simulink model "Launch_controlV1_a"  (R2015a)
settings: Solver=ode3  StartTime=0.0  StopTime=inf  FixedStep=0.001  RelTol=1e-3
undefined symbols (not defined in the file or in its folder): DiscIntNeverNeededParam, Ts
libraries: simulink x3
settings Model: CovModelRefEnable=off  Creator=Sven-VDR  LastModifiedBy=Sven-VDR
settings DataIOCC: SaveFormat=Dataset
settings HardwareCC: ProdBitPerPointer=64  ProdLargestAtomicFloat=Float  ProdIntDivRoundTo=Zero  ProdEndianess=LittleEndian  ProdHWDeviceType=Specified
settings GRTTargetCC: GeneratePreprocessorConditionals=Use local settings

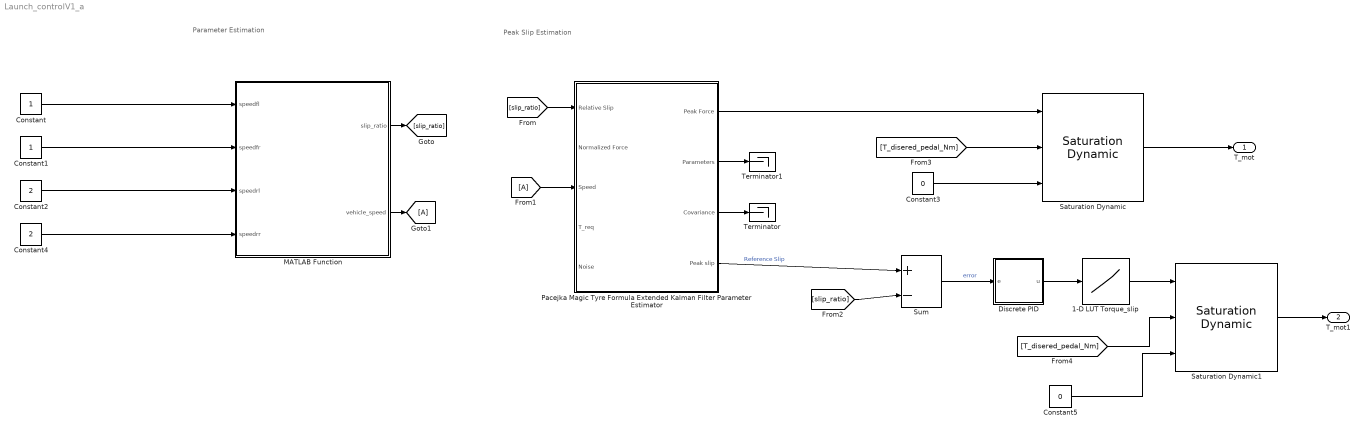
== system Launch_controlV1_a ==
  note: Peak Slip Estimation
  note: Parameter Estimation
  1-D LUT Torque_slip : Lookup_n-D  NumberOfTableDimensions=1  BreakpointsForDimension1=[-5:5]  Table=tanh([-5:5])  InternalRulePriority=Speed  RndMeth=Simplest  InputSameDT=on
  Constant : Constant
  Constant1 : Constant
  Constant2 : Constant  Value=2
  Constant3 : Constant  Value=0
  Constant4 : Constant  Value=2
  Constant5 : Constant  Value=0
  Discrete PID : Subsystem
  MATLAB Function : MATLAB Function  TreatAsAtomicUnit=on
      settings: PermitHierarchicalResolution=ParametersOnly
  Pacejka Magic Tyre Formula Extended Kalman Filter Parameter Estimator : Subsystem
  Saturation Dynamic : simulink/Discontinuities/Saturation Dynamic  OutMin=[]  OutMax=[]  OutDataTypeStr=Inherit: Same as second input  OutDataType=fixdt(1, 16)  OutScaling=2^-10  DoSatur=off
  Saturation Dynamic1 : simulink/Discontinuities/Saturation Dynamic  OutMin=[]  OutMax=[]  OutDataTypeStr=Inherit: Same as second input  OutDataType=fixdt(1, 16)  OutScaling=2^-10  DoSatur=off
  Sum : Sum  Inputs=+|-
  Terminator : Terminator
  Terminator1 : Terminator
  T_mot : Outport
  T_mot1 : Outport  Port=2
  wires:
  Constant2/1 -> MATLAB Function/3(speedrl)
  Constant/1 -> MATLAB Function/1(speedfl)
  Constant4/1 -> MATLAB Function/4(speedrr)
  Constant1/1 -> MATLAB Function/2(speedfr)
  MATLAB Function/1(slip_ratio) -> [slip_ratio]
  MATLAB Function/2(vehicle_speed) -> [A]
  [slip_ratio] -> Pacejka Magic Tyre Formula Extended Kalman Filter Parameter Estimator/1(Relative Slip)
  [A] -> Pacejka Magic Tyre Formula Extended Kalman Filter Parameter Estimator/3(Speed)
  Pacejka Magic Tyre Formula Extended Kalman Filter Parameter Estimator/4(Peak slip) -> Sum/1  "Reference Slip"
  Pacejka Magic Tyre Formula Extended Kalman Filter Parameter Estimator/3(Covariance) -> Terminator/1
  Pacejka Magic Tyre Formula Extended Kalman Filter Parameter Estimator/2(Parameters) -> Terminator1/1
  Sum/1 -> Discrete PID/1("e ")  "error"
  [slip_ratio] -> Sum/2
  Constant3/1 -> Saturation Dynamic/3
  Pacejka Magic Tyre Formula Extended Kalman Filter Parameter Estimator/1(Peak Force) -> Saturation Dynamic/1
  [T_disered_pedal_Nm] -> Saturation Dynamic/2
  Saturation Dynamic/1 -> T_mot/1
  Discrete PID/1(u) -> 1-D LUT Torque_slip/1
  1-D LUT Torque_slip/1 -> Saturation Dynamic1/1
  [T_disered_pedal_Nm] -> Saturation Dynamic1/2
  Constant5/1 -> Saturation Dynamic1/3
  Saturation Dynamic1/1 -> T_mot1/1

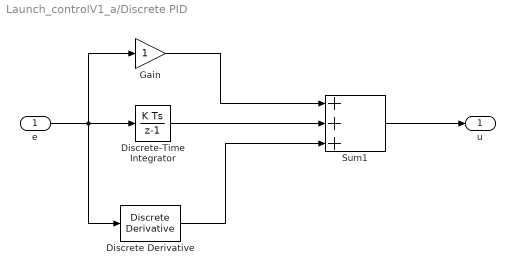
== system Launch_controlV1_a/Discrete PID ==
  "e " : Inport
  Discrete Derivative : simulink/Discrete/Discrete Derivative  gainval=1.0  ICPrevScaledInput=0.0  InputProcessing=Inherited  OutMin=[]  OutMax=[]  OutDataType=fixdt(1, 16)  OutScaling=2^-10  DoSatur=off
  Discrete-Time Integrator : DiscreteIntegrator  InitialConditionSetting=State (most efficient)  ICPrevOutput=DiscIntNeverNeededParam  ICPrevScaledInput=DiscIntNeverNeededParam
  Gain : Gain
  Sum1 : Sum  Inputs=+|+|+
  u : Outport
  wires:
  "e "/1 -> Discrete Derivative/1, Discrete-Time Integrator/1, Gain/1
  Sum1/1 -> u/1
  Discrete-Time Integrator/1 -> Sum1/2
  Gain/1 -> Sum1/1
  Discrete Derivative/1 -> Sum1/3

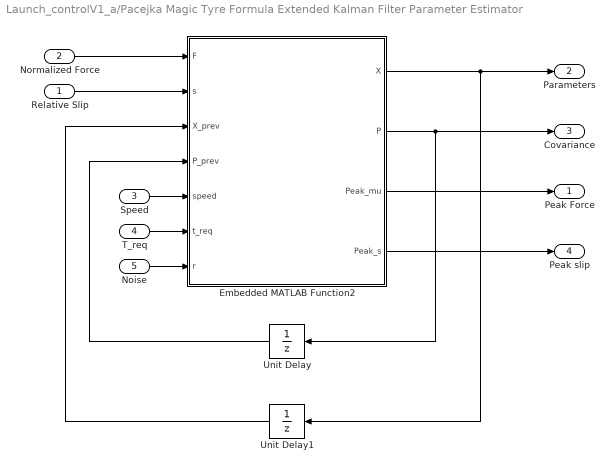
== system Launch_controlV1_a/Pacejka Magic Tyre Formula Extended Kalman Filter Parameter Estimator ==
  Relative Slip : Inport
  Normalized Force : Inport  Port=2
  Speed : Inport  Port=3
  T_req : Inport  Port=4
  Noise : Inport  Port=5
  Embedded MATLAB Function2 : MATLAB Function  TreatAsAtomicUnit=on
      settings: PermitHierarchicalResolution=ParametersOnly
  Unit Delay : UnitDelay  InitialCondition=[1 0 0 0 0; 0 3 0 0 0; 0 0 3 0 0; 0 0 0 0.5 0; 0 0 0 0 5]  SampleTime=Ts
  Unit Delay1 : UnitDelay  InitialCondition=[15;2;2;0.9;0]  SampleTime=Ts
  Peak Force : Outport
  Parameters : Outport  Port=2
  Covariance : Outport  Port=3
  Peak slip : Outport  Port=4
  wires:
  Embedded MATLAB Function2/2(P) -> Covariance/1, Unit Delay/1
  Unit Delay/1 -> Embedded MATLAB Function2/4(P_prev)
  Embedded MATLAB Function2/1(X) -> Parameters/1, Unit Delay1/1
  Unit Delay1/1 -> Embedded MATLAB Function2/3(X_prev)
  Normalized Force/1 -> Embedded MATLAB Function2/1(F)
  Relative Slip/1 -> Embedded MATLAB Function2/2(s)
  Embedded MATLAB Function2/3(Peak_mu) -> Peak Force/1
  Speed/1 -> Embedded MATLAB Function2/5(speed)
  T_req/1 -> Embedded MATLAB Function2/6(t_req)
  Noise/1 -> Embedded MATLAB Function2/7(r)
  Embedded MATLAB Function2/4(Peak_s) -> Peak slip/1

== matlab function Launch_controlV1_a/MATLAB Function ==
  data: speedfl input; slip_ratio output; speedfr input; speedrl input; speedrr input; vehicle_speed output
function [slip_ratio, vehicle_speed]=Launch_slip_calc(speedfl,speedfr,speedrl,speedrr)
%Calculates the wheel slip ratio
rwheel=0.254; %m

Rotspeed_front=(speedfl+speedfr)/2;
Rotspeed_rear = max(speedrl,speedrr);

vehicle_speed=Rotspeed_front*rwheel;

slip_ratio=(1-vehicle_speed/(rwheel*Rotspeed_rear));

if slip_ratio<0
    slip_ratio=0;
end

end

== matlab function Launch_controlV1_a/Pacejka Magic Tyre Formula Extended Kalman Filter Parameter Estimator/Embedded MATLAB Function2 ==
  data: F input; s input; X_prev input; X output; P_prev input; P output; Peak_mu output; speed input; t_req input; r input; Peak_s output
function [X,P,Peak_mu,Peak_s]= Magic_Formula(F,s,X_prev,P_prev,speed,t_req,r)
    
% Initialization

X = X_prev;
P = P_prev;

% Kalman Filter Algorithm (Pacejka Magic Formula)
% State X consists of B, C, D, E, Sv, Sh (in this order)

B = X(1,1);
C = X(2,1);
D = X(3,1);
E = X(4,1);
Sh = X(5,1);

% Noise
%r = [0.01 0; 0 0.1];

if (s >= 0.02 && s <= 0.10 && F >= 0.5 && speed >= 10 && t_req >= 50)
    
% Define a,b,c and d to make my life a lot easier

a = D*cos(C*atan(-B*(s+Sh)+E*(B*(s+Sh)-atan(B*(s+Sh)))));
b = 1+(-B*(s+Sh)+E*(B*(s+Sh)-atan(B*(s+Sh))))^2;
c = s+Sh;
d = 1+(B^2)*(s+Sh)^2;

% The h matrix

h = [(a*C*(-c+E*(c-(c/d))))/b a*atan(-B*c+E*(B*c-atan(B*c))) sin(C*atan(-B*c+E*(B*c-atan(B*c)))) a*C*(B*c-atan(B*c))/b a*C*(-B+E*(B-(B/(1+(B^2)*(c^2)))))/b];

% The v matrix

v = [1 (a*C*(-B+E*(B-(B/(1+(B^2)*(c^2))))))/b];

% K matrix

K = P*transpose(h)*((h*P*transpose(h))+(v*r*transpose(v)))^-1;

P = (eye(5)-K*h)*P;

X = X + K*(-F+D*sin(C*atan(B*c-E*(B*c-atan(B*c)))));

if (X(4,1) >= 1)
    X(4,1) = 1;
end
    

end

Peak_mu = X(3,1);

Peak_s = (0.5099439062*10^-4)*sqrt((2.5*10^9)-(4.78*10^8)*X(4,1)+(1.6476597*10^8)*(X(4,1)^2)-(1.961*10^9)*X(4,1)*tan(1.570796327/X(2,1)))/(X(4,1)*X(1,1))
